simulink model "DualStreamSSR"  (R2020a)
settings: Solver=VariableStepAuto  StartTime=0.0  StopTime=4096  RelTol=1e-3
PreLoadFcn:
  | SSR4_init
InitFcn:
  | SSR4_init
values from neighbouring files (symbols this model uses):
  N = 8    [SSR4_init.m]
  SHIFT_ACC = 15    [SSR4_init.m]
  Taps = NormalizeCoef(UTaps,32768)    [SSR4_init.m]
undefined symbols (not defined in the file or in its folder): DoubleStream, FIR_MultiKernel_cin, FIR_MultiKernel_cincout, FIR_MultiKernel_cout, xc7vx485tffg1157
libraries: ModelComposer x129, dspsrcs4 x1, simulink x1
(part 1 of 5)
settings Model: PauseTimes=120  NumberOfSteps=64  Creator=viswanad  LastModifiedBy=viswanad

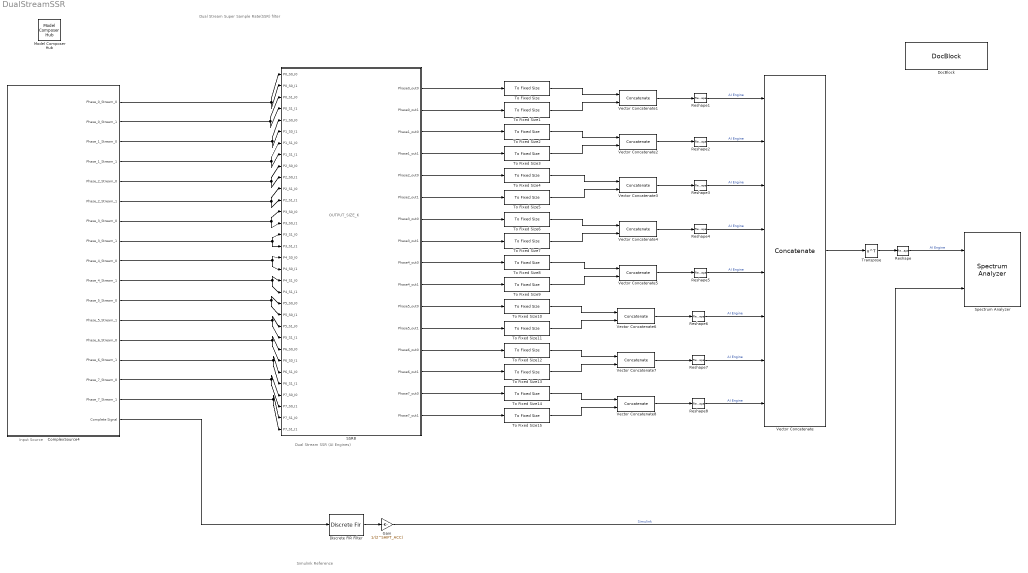
== system DualStreamSSR ==
  note: Dual Stream SSR
      | (AI Engines)
  note: OUTPUT_SIZE_K
  note: Dual Stream Super Sample Rate(SSR) filter
  note: Simulink Reference
  note: Input Source
  ComplexSource4 : Subsystem  mask{s=0}
      mask prompts: s "Seed"
  Discrete FIR Filter : DiscreteFir  Coefficients=Taps  InputProcessing=Columns as channels (frame based)
  DocBlock : simulink/Model-Wide Utilities/DocBlock  DocumentType=Text  mask(DocBlock){}
      content=|
      | ///////////////////////////////////////////////////////////////////////////
      | // Copyright 2021 Xilinx
      | //
      | // Licensed under the Apache License, Version 2.0 (the "License");
      | // you may not use this file except in compliance with the License.
      | // You may obtain a copy of the License at
      | //
      | // http://www.apache.org/licenses/LICENSE-2.0
      | //
      | // Unless required by applicable law or agreed to in writing, software
      | // distributed under the License is distributed on an "AS IS" BASIS,
      | // WITHOUT WARRANTIES OR CONDITIONS OF ANY KIND, either express or implied.
      | // See the License for the specific language governing permissions and
      | // limitations under the License.
      | ///////////////////////////////////////////////////////////////////////////
      mask Display:
      | xmcDrawBlockIcon();
      | disp(['{\fontsize{10pt}(c) Copyright 2021' ' Xilinx, Inc.}\newline \newline '],'texmode','on');
      | disp('{\fontsize{10pt}Licensed under the Apache License 2.0}','texmode','on');
      | disp('\newline \newline \newline{\fontsize{10pt}Double Click for Copyright Notice}','texmode','on');
  Gain : Gain  Gain=1/(2^SHIFT_ACC)
  Model Composer Hub : ModelComposer/Model Composer Hub  CodeGeneration=off  SubsystemName=SSR8  TargetDirectory=./code  ExportType=AI Engines  IpVendor=xilinx.com  IpLibrary=hls  IpVersion=1.0  IpHWLanguage=Verilog  AieCompilerOptions={}  CreateTestbench=on  TestbenchStackSize=10  RunAieSim=on  AieSimTimeout=50000  RunAieSimProfiling=off  LaunchVitisAnalyzer=off  PlotOutput=on  RunX86Sim=off  X86SimTimeout=10  GenHwImage=off  PlatformType=Not Specified  ProjDevice=xc7vx485tffg1157-1  ProjDevicePart=xc7vx485tffg1157-1  SamplePeriod=-1  ClockFrequency=200  DataPathParallelism=1
  Reshape{,1..8} (9 alike) : Reshape
  SSR8 : Subsystem
  Spectrum Analyzer : SpectrumAnalyzer  NumInputPorts=2
  To Fixed Size{,1..15} (16 alike) : ModelComposer/To Fixed Size  OutputSize=Inherit: Same as input  CopyMethod=Pad with zeros or discard excess samples (WILL BE DEPRECATED)  HasStatusOutput=off
  Transpose : Math  Operator=transpose  SaturateOnIntegerOverflow=on
  Vector Concatenate : Concatenate  NumInputs=8  Mode=Multidimensional array  ConcatenateDimension=2
  Vector Concatenate{1..8} (8 alike) : Concatenate  Mode=Multidimensional array
  wires:
  ComplexSource4/1(Phase_0_Stream_0) -> SSR8/1(P0_S0_I0), SSR8/2(P0_S0_I1)
  ComplexSource4/2(Phase_0_Stream_1) -> SSR8/3(P0_S1_I0), SSR8/4(P0_S1_I1)
  ComplexSource4/3(Phase_1_Stream_0) -> SSR8/5(P1_S0_I0), SSR8/6(P1_S0_I1)
  ComplexSource4/4(Phase_1_Stream_1) -> SSR8/8(P1_S1_I1), SSR8/7(P1_S1_I0)
  ComplexSource4/5(Phase_2_Stream_0) -> SSR8/10(P2_S0_I1), SSR8/9(P2_S0_I0)
  ComplexSource4/6(Phase_2_Stream_1) -> SSR8/12(P2_S1_I1), SSR8/11(P2_S1_I0)
  ComplexSource4/7(Phase_3_Stream_0) -> SSR8/14(P3_S0_I1), SSR8/13(P3_S0_I0)
  ComplexSource4/8(Phase_3_Stream_1) -> SSR8/16(P3_S1_I1), SSR8/15(P3_S1_I0)
  ComplexSource4/9(Phase_4_Stream_0) -> SSR8/18(P4_S0_I1), SSR8/17(P4_S0_I0)
  ComplexSource4/10(Phase_4_Stream_1) -> SSR8/20(P4_S1_I1), SSR8/19(P4_S1_I0)
  ComplexSource4/11(Phase_5_Stream_0) -> SSR8/22(P5_S0_I1), SSR8/21(P5_S0_I0)
  ComplexSource4/12(Phase_5_Stream_1) -> SSR8/24(P5_S1_I1), SSR8/23(P5_S1_I0)
  ComplexSource4/13(Phase_6_Stream_0) -> SSR8/26(P6_S0_I1), SSR8/25(P6_S0_I0)
  ComplexSource4/14(Phase_6_Stream_1) -> SSR8/28(P6_S1_I1), SSR8/27(P6_S1_I0)
  ComplexSource4/15(Phase_7_Stream_0) -> SSR8/30(P7_S0_I1), SSR8/29(P7_S0_I0)
  ComplexSource4/16(Phase_7_Stream_1) -> SSR8/32(P7_S1_I1), SSR8/31(P7_S1_I0)
  Discrete FIR Filter/1 -> Gain/1
  ComplexSource4/17(Complete Signal) -> Discrete FIR Filter/1
  Transpose/1 -> Reshape/1
  Vector Concatenate/1 -> Transpose/1
  Reshape/1 -> Spectrum Analyzer/1  "AI Engine"
  SSR8/1(Phase0_out0) -> To Fixed Size/1
  To Fixed Size/1 -> Vector Concatenate1/1
  SSR8/2(Phase0_out1) -> To Fixed Size1/1
  SSR8/3(Phase1_out0) -> To Fixed Size2/1
  SSR8/4(Phase1_out1) -> To Fixed Size3/1
  SSR8/5(Phase2_out0) -> To Fixed Size4/1
  SSR8/6(Phase2_out1) -> To Fixed Size5/1
  SSR8/7(Phase3_out0) -> To Fixed Size6/1
  SSR8/8(Phase3_out1) -> To Fixed Size7/1
  SSR8/9(Phase4_out0) -> To Fixed Size8/1
  SSR8/10(Phase4_out1) -> To Fixed Size9/1
  SSR8/11(Phase5_out0) -> To Fixed Size10/1
  SSR8/12(Phase5_out1) -> To Fixed Size11/1
  SSR8/13(Phase6_out0) -> To Fixed Size12/1
  SSR8/14(Phase6_out1) -> To Fixed Size13/1
  SSR8/15(Phase7_out0) -> To Fixed Size14/1
  SSR8/16(Phase7_out1) -> To Fixed Size15/1
  To Fixed Size1/1 -> Vector Concatenate1/2
  Vector Concatenate1/1 -> Reshape1/1
  Vector Concatenate2/1 -> Reshape2/1
  Vector Concatenate3/1 -> Reshape3/1
  Vector Concatenate4/1 -> Reshape4/1
  Vector Concatenate5/1 -> Reshape5/1
  Vector Concatenate6/1 -> Reshape6/1
  Vector Concatenate7/1 -> Reshape7/1
  Vector Concatenate8/1 -> Reshape8/1
  To Fixed Size2/1 -> Vector Concatenate2/1
  To Fixed Size3/1 -> Vector Concatenate2/2
  To Fixed Size4/1 -> Vector Concatenate3/1
  To Fixed Size5/1 -> Vector Concatenate3/2
  To Fixed Size6/1 -> Vector Concatenate4/1
  To Fixed Size7/1 -> Vector Concatenate4/2
  To Fixed Size8/1 -> Vector Concatenate5/1
  To Fixed Size9/1 -> Vector Concatenate5/2
  To Fixed Size10/1 -> Vector Concatenate6/1
  To Fixed Size11/1 -> Vector Concatenate6/2
  To Fixed Size12/1 -> Vector Concatenate7/1
  To Fixed Size13/1 -> Vector Concatenate7/2
  To Fixed Size14/1 -> Vector Concatenate8/1
  To Fixed Size15/1 -> Vector Concatenate8/2
  Reshape1/1 -> Vector Concatenate/1  "AI Engine"
  Reshape2/1 -> Vector Concatenate/2  "AI Engine"
  Reshape3/1 -> Vector Concatenate/3  "AI Engine"
  Reshape4/1 -> Vector Concatenate/4  "AI Engine"
  Reshape5/1 -> Vector Concatenate/5  "AI Engine"
  Reshape6/1 -> Vector Concatenate/6  "AI Engine"
  Reshape7/1 -> Vector Concatenate/7  "AI Engine"
  Reshape8/1 -> Vector Concatenate/8  "AI Engine"
  Gain/1 -> Spectrum Analyzer/2  "Simulink"

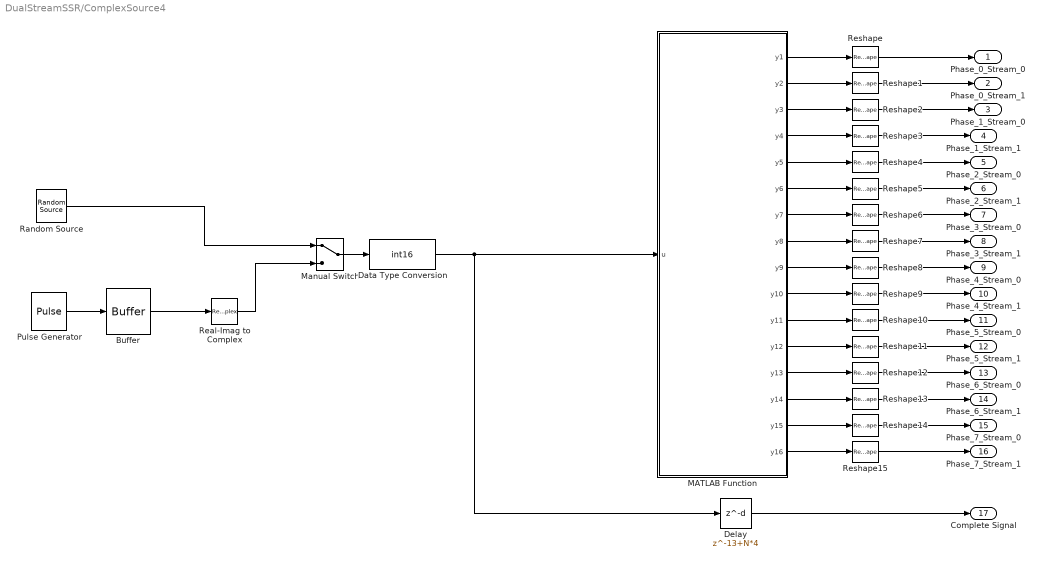
== system DualStreamSSR/ComplexSource4 ==
  Buffer : Buffer  N=N*8  OutputFrames=off
  Data Type Conversion : DataTypeConversion  OutDataTypeStr=int16
  Delay : Delay  DelayLength=13+N*4  InputProcessing=Columns as channels (frame based)
  MATLAB Function : MATLAB Function  TreatAsAtomicUnit=on
  Manual Switch : ManualSwitch
  Pulse Generator : DiscretePulseGenerator  Amplitude=20000  Period=32 + 40*5  PhaseDelay=32  SampleTime=1/8
  Random Source : dspsrcs4/Random Source  SrcType=Uniform  NormMethod=Ziggurat  CltLength=12  MinVal=-20000  MaxVal=20000  MeanVal=0  VarVal=1  RepMode=Specify seed  rawSeed=s  IsInherit=off  SampMode=Discrete  SampTime=1/8  SampFrame=8*N  DataType=Double  OutComplex=Complex  OutputFrames=off
  Real-Imag to Complex : RealImagToComplex  Input=Real
  Reshape{,1..15} (16 alike) : Reshape
  Phase_0_Stream_0 : Outport
  Phase_0_Stream_1 : Outport  Port=2
  Phase_1_Stream_0 : Outport  Port=3
  Phase_1_Stream_1 : Outport  Port=4
  Phase_2_Stream_0 : Outport  Port=5
  Phase_2_Stream_1 : Outport  Port=6
  Phase_3_Stream_0 : Outport  Port=7
  Phase_3_Stream_1 : Outport  Port=8
  Phase_4_Stream_0 : Outport  Port=9
  Phase_4_Stream_1 : Outport  Port=10
  Phase_5_Stream_0 : Outport  Port=11
  Phase_5_Stream_1 : Outport  Port=12
  Phase_6_Stream_0 : Outport  Port=13
  Phase_6_Stream_1 : Outport  Port=14
  Phase_7_Stream_0 : Outport  Port=15
  Phase_7_Stream_1 : Outport  Port=16
  Complete Signal : Outport  Port=17
  wires:
  MATLAB Function/1(y1) -> Reshape/1
  MATLAB Function/2(y2) -> Reshape1/1
  MATLAB Function/3(y3) -> Reshape2/1
  MATLAB Function/4(y4) -> Reshape3/1
  Real-Imag to Complex/1 -> Manual Switch/2
  Pulse Generator/1 -> Buffer/1
  Delay/1 -> Complete Signal/1
  Buffer/1 -> Real-Imag to Complex/1
  Manual Switch/1 -> Data Type Conversion/1
  MATLAB Function/5(y5) -> Reshape4/1
  MATLAB Function/6(y6) -> Reshape5/1
  MATLAB Function/7(y7) -> Reshape6/1
  MATLAB Function/8(y8) -> Reshape7/1
  MATLAB Function/9(y9) -> Reshape8/1
  MATLAB Function/10(y10) -> Reshape9/1
  MATLAB Function/11(y11) -> Reshape10/1
  MATLAB Function/12(y12) -> Reshape11/1
  MATLAB Function/13(y13) -> Reshape12/1
  MATLAB Function/14(y14) -> Reshape13/1
  MATLAB Function/15(y15) -> Reshape14/1
  MATLAB Function/16(y16) -> Reshape15/1
  Data Type Conversion/1 -> MATLAB Function/1(u), Delay/1
  Reshape/1 -> Phase_0_Stream_0/1
  Reshape1/1 -> Phase_0_Stream_1/1
  Reshape2/1 -> Phase_1_Stream_0/1
  Reshape3/1 -> Phase_1_Stream_1/1
  Reshape4/1 -> Phase_2_Stream_0/1
  Reshape5/1 -> Phase_2_Stream_1/1
  Reshape6/1 -> Phase_3_Stream_0/1
  Reshape7/1 -> Phase_3_Stream_1/1
  Reshape8/1 -> Phase_4_Stream_0/1
  Reshape9/1 -> Phase_4_Stream_1/1
  Reshape10/1 -> Phase_5_Stream_0/1
  Reshape11/1 -> Phase_5_Stream_1/1
  Reshape12/1 -> Phase_6_Stream_0/1
  Reshape13/1 -> Phase_6_Stream_1/1
  Reshape14/1 -> Phase_7_Stream_0/1
  Reshape15/1 -> Phase_7_Stream_1/1
  Random Source/1 -> Manual Switch/1
